simulink model "AllPassInst"  (R2016b)
settings: Solver=ode45  StartTime=0.0  StopTime=.75  RelTol=1e-10  EnableMultiTasking=on
settings Model: Creator=Adolfo  LastModifiedBy=adolfobs
settings SolverCC: ConsecutiveZCsStepRelTol=eps
settings DataIOCC: LimitDataPoints=on  SaveFormat=Array  SignalLoggingSaveFormat=ModelDataLogs
settings OptimizationCC: ExpressionDepthLimit=2147483647  LifeSpan=inf
settings DebuggingCC: UnderspecifiedInitializationDetection=Classic  MergeDetectMultiDrivingBlocksExec=none  SolverPrmCheckMsg=warning  FcnCallInpInsideContextMsg=warning  StateNameClashWarn=warning  SFUnexpectedBacktrackingDiag=warning  SFNoUnconditionalDefaultTransitionDiag=warning  SFExecutionAtInitializationDiag=none
settings HardwareCC: ProdBitPerPointer=32  ProdBitPerSizeT=32  ProdBitPerPtrDiffT=32  ProdLargestAtomicFloat=None  ProdIntDivRoundTo=Undefined  ProdEndianess=Unspecified  ProdWordSize=32  ProdHWDeviceType=32-bit Generic
settings ModelReferenceCC: PropagateSignalLabelsOutOfModel=off
settings GRTTargetCC: TargetLangStandard=C89/C90 (ANSI)  GeneratePreprocessorConditionals=Disable all  CombineOutputUpdateFcns=off  GRTInterface=on
settings ConfigComp: CovMetricSettings=dw  CovHtmlReporting=on  CovSaveCumulativeToWorkspaceVar=on  CovSaveSingleToWorkspaceVar=on  CovExternalEMLEnable=off

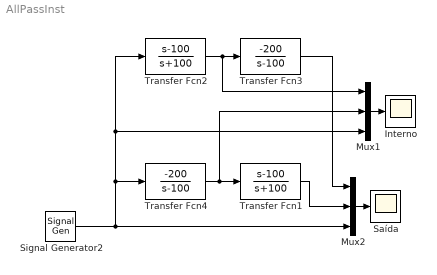
== system AllPassInst ==
  Interno : Scope
  Mux1 : Mux  Inputs=3
  Mux2 : Mux  Inputs=3
  Saída : Scope
  Signal Generator2 : SignalGenerator  WaveForm=square  Frequency=10
  Transfer Fcn1 : TransferFcn  Numerator=[1 -100]  Denominator=[1 100]
  Transfer Fcn2 : TransferFcn  Numerator=[1 -100]  Denominator=[1 100]
  Transfer Fcn3 : TransferFcn  Numerator=[-200]  Denominator=[1 -100]
  Transfer Fcn4 : TransferFcn  Numerator=[-200]  Denominator=[1 -100]
  wires:
  Mux2/1 -> Saída/1
  Signal Generator2/1 -> Transfer Fcn2/1, Mux1/3, Transfer Fcn4/1, Mux2/3
  Transfer Fcn2/1 -> Mux1/1, Transfer Fcn3/1
  Mux1/1 -> Interno/1
  Transfer Fcn4/1 -> Mux1/2, Transfer Fcn1/1
  Transfer Fcn3/1 -> Mux2/1
  Transfer Fcn1/1 -> Mux2/2
